simulink model "MSE_312_Electrical_Control_Model_The_Iron_Pirate"  (R2021a)
settings: Solver=ode15s  StartTime=0.0  StopTime=35  MaxStep=1  RelTol=1e-4  AbsTol=1e-4
libraries: fl_lib x15, nesl_utility x11, ee_lib x3, pid_lib x2
settings Model: Creator=junaidkhan  LastModifiedBy=Imad

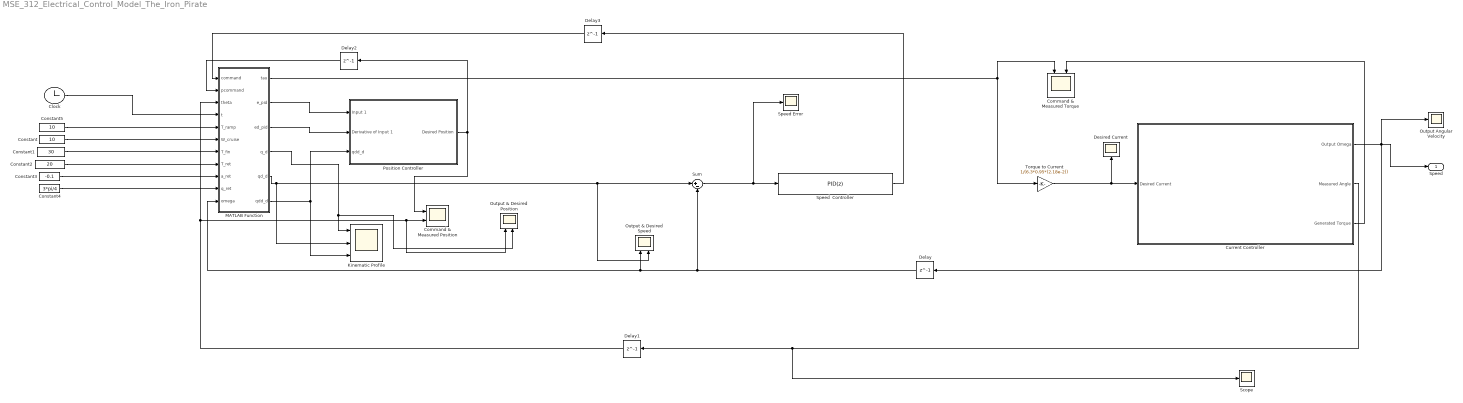
== system MSE_312_Electrical_Control_Model_The_Iron_Pirate ==
  " Output Angular Velocity" : Scope
  Clock : Clock
  Command & Measured Position : Scope  NumInputPorts=2
  Command & Measured Torque : Scope  NumInputPorts=2
  Constant : Constant  Value=10
  Constant1 : Constant  Value=30
  Constant2 : Constant  Value=20
  Constant3 : Constant  Value=-0.1
  Constant4 : Constant  Value=3*pi/4
  Constant5 : Constant  Value=10
  Current Controller : Subsystem
  Delay{,1..3} (4 alike) : Delay  DelayLength=1
  Desired Current : Scope
  Kinematic Profile : Scope  NumInputPorts=3
  MATLAB Function : MATLAB Function  TreatAsAtomicUnit=on
  Output & Desired Position : Scope  NumInputPorts=2
  Output & Desired Speed : Scope  NumInputPorts=2
  "Position Controller " : Subsystem
  Scope : Scope
  Speed  Controller : pid_lib/PID Controller  Controller=PID  Form=Ideal  TimeDomain=Discrete-time  UseExternalTs=off  SampleTime=1/4000  IntegratorMethod=Forward Euler  FilterMethod=Forward Euler  ControllerParametersSource=internal  P=1200*(0.00234)*(1/10)  I=0.0132  D=0.001  UseFilter=on  N=100  TunerSelectOption=Frequency Response Based  InitialConditionSource=internal  InitialConditionForIntegrator=0  InitialConditionForFilter=0  DifferentiatorICPrevScaledInput=0  ExternalReset=none  TrackingMode=off  Kt=1  LimitOutput=off  SatLimitsSource=internal  UpperSaturationLimit=inf  LowerSaturationLimit=-inf  LinearizeAsGain=on  AntiWindupMode=none  Kb=1  POutMin=[]  POutMax=[]  IOutMin=[]  IOutMax=[]  DOutMin=[]  DOutMax=[]  NOutMin=[]  NOutMax=[]  SumOutMin=[]  SumOutMax=[]  SaturationOutMin=[]  SaturationOutMax=[]  PParamMin=[]  PParamMax=[]  IParamMin=[]  IParamMax=[]  DParamMin=[]  DParamMax=[]  NParamMin=[]  NParamMax=[]  KbParamMin=[]  KbParamMax=[]  KtParamMin=[]  KtParamMax=[]  KbOutMin=[]  KbOutMax=[]  KtOutMin=[]  KtOutMax=[]  IntegratorOutMin=[]  IntegratorOutMax=[]  FilterOutMin=[]  FilterOutMax=[]  SumI1OutMin=[]  SumI1OutMax=[]  SumI2OutMin=[]  SumI2OutMax=[]  SumI3OutMin=[]  SumI3OutMax=[]  SumI4OutMin=[]  SumI4OutMax=[]  SumDOutMin=[]  SumDOutMax=[]  DifferentiatorOutMin=[]  DifferentiatorOutMax=[]  FilterDiffOutCoefMin=[]  FilterDiffOutCoefMax=[]  ReciprocalOutMin=[]  ReciprocalOutMax=[]  SumDenOutMin=[]  SumDenOutMax=[]  SumNumOutMin=[]  SumNumOutMax=[]  DivideOutMin=[]  DivideOutMax=[]  UdiffTsProdOutMin=[]  UdiffTsProdOutMax=[]  NTsProdOutMin=[]  NTsProdOutMax=[]  UintegralTsProdOutMin=[]  UintegralTsProdOutMax=[]  UngainTsProdOutMin=[]  UngainTsProdOutMax=[]  IntegratorContinuousStateAttributes=''  IntegratorStateMustResolveToSignalObject=off  IntegratorRTWStateStorageClass=Auto  FilterContinuousStateAttributes=''  FilterStateMustResolveToSignalObject=off  FilterRTWStateStorageClass=Auto  ParallelPVariant=Passthrough  IdealPVariant=InternalParameters  IVariant=InternalParameters  DVariant=InternalParameters  IntegratorVariant=Discrete  SatVariant=Disabled  AWVariant=Passthrough  PCopyVariant=Disabled  TRVariant=Disabled  FdbkBlocksVariant=Forward  IdealPFdbkVariant=Disabled  SatFdbkVariant=Disabled  DerivativeFilterVariant=ForwardEulerFilter  NVariant=InternalParameters  NCopyVariant=Disabled  FilterICVariant=InternalICsFilter  IntegratorICVariant=InternalICs  ExternalResetVariant=Disabled  TRSumVariant=Passthrough  SumFdbkVariant=Disabled  SumVariant=Sum_PID  TsampFilterVariant=InternalTs  TsampNgainVariant=Passthrough  TsampIntegralVariant=Passthrough  ExternalSaturationOutDataTypeStr=Inherit: Same as second input
  Speed Error : Scope
  Sum : Sum  Inputs=|+-
  Torque to Current : Gain  Gain=1/(6.3*0.95*(2.18e-2))
  Speed : Outport
  wires:
  Torque to Current/1 -> Current Controller/1("Desired Current "), Desired Current/1
  Speed  Controller/1 -> Delay3/1
  Sum/1 -> Speed Error/1, Speed  Controller/1
  Current Controller/3(Generated Torque) -> Command & Measured Torque/2
  MATLAB Function/5(qd_d) -> Sum/1, Output & Desired Speed/2, Kinematic Profile/2
  Delay/1 -> Sum/2, Output & Desired Speed/1, MATLAB Function/11(omega)
  Clock/1 -> MATLAB Function/4(t)
  Constant2/1 -> MATLAB Function/8(T_ret)
  Constant5/1 -> MATLAB Function/5(T_ramp)
  Constant3/1 -> MATLAB Function/9(a_ret)
  Constant4/1 -> MATLAB Function/10(q_ret)
  Constant/1 -> MATLAB Function/6(W_cruise)
  Constant1/1 -> MATLAB Function/7(T_fin)
  MATLAB Function/1(tau) -> Torque to Current/1, Command & Measured Torque/1
  Delay1/1 -> MATLAB Function/3(theta), Output & Desired Position/1, Command & Measured Position/2
  MATLAB Function/2(e_pid) -> "Position Controller "/1(Input 1)
  MATLAB Function/3(ed_pid) -> "Position Controller "/2(Derivative of Input 1)
  MATLAB Function/6(qdd_d) -> Kinematic Profile/3, "Position Controller "/3(qdd_d)
  MATLAB Function/4(q_d) -> Output & Desired Position/2, Kinematic Profile/1
  "Position Controller "/1(Desired Position) -> Command & Measured Position/1, Delay2/1
  Current Controller/1(Output Omega) -> Delay/1, Speed/1, " Output Angular Velocity"/1
  Current Controller/2("Measured Angle ") -> Scope/1, Delay1/1
  Delay2/1 -> MATLAB Function/2(pcommand)
  Delay3/1 -> MATLAB Function/1(command)

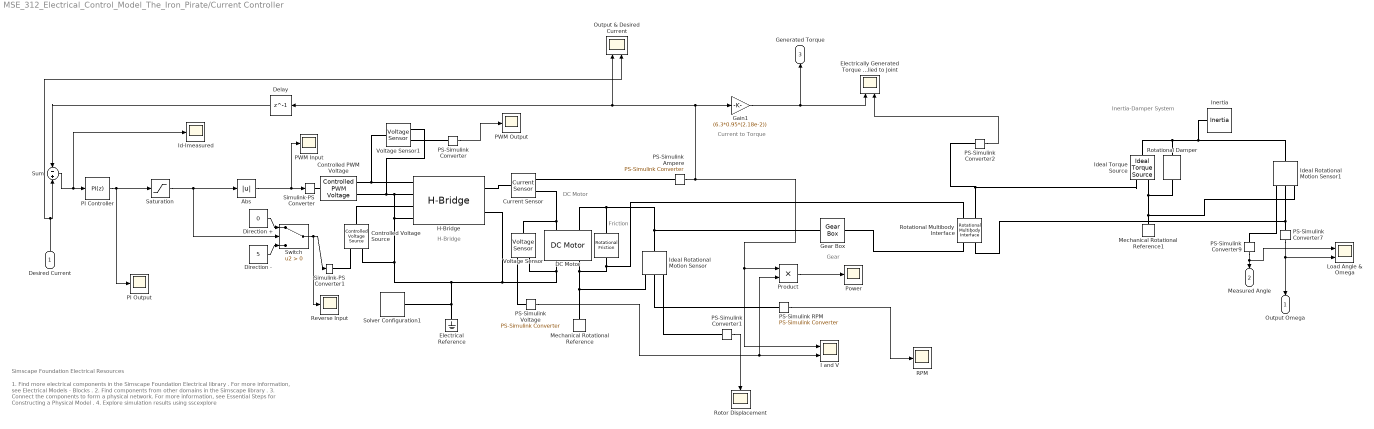
== system MSE_312_Electrical_Control_Model_The_Iron_Pirate/Current Controller ==
  note: Inertia-Damper System
  note: Current to Torque
  note: Gear
  note: H-Bridge
  note: DC Motor
  note: Friction
  note: 1. Find more electrical components in the Simscape Foundation Electrical library .
      | For more information, see Electrical Models - Blocks .
      | 2. Find components from other domains in the Simscape library .
      | 3. Connect the components to form a physical network.
      | For more information, see Essential Steps for Constructing a Physical Model .
      | 4. Explore simulation results using sscexplore
  note: Simscape Foundation Electrical Resources
  "Desired Current " : Inport
  " " : fl_lib/Mechanical/Rotational Elements/Rotational Friction  brkwy_trq=2.5e-3 N*m  brkwy_vel=0.1 rad/s  Col_trq=2.5e-3 N*m  visc_coef=0.001 N*m/(rad/s)  w_specify=off  w_priority=None  w=0 rad/s  w_nominal_specify=off  w_nominal_unit=rad/s  w_nominal_value=1  t_specify=off  t_priority=None  t=0 N*m  t_nominal_specify=off  t_nominal_unit=N*m  t_nominal_value=1
  Abs : Abs
  Controlled PWM Voltage : ee_lib/Integrated Circuits/Controlled PWM Voltage  F=4000 Hz  TD=0 s  pulse_width_offset=0 s  pulse_min=1 us  Vmin=0 V  Vmax=12 V  Vm=12 V  pwm_or_av=2  event_type=1  sample_time=1e-6 s  u_min=0  u_max=12
      settings: InternalSimscapePortConfiguration="{\"Bottom\":[],\"Left\":[{\"id\":\"u\",\"label\":\"u\",\"type\":\"input\"}],\"Right\":[{\"id\":\"p2\",\"label\":\"PWM\",\"type\":\"foundation.electrical.electrical\"},{\"id\":\"n2\",\"label\":\"REF\",\"type\":\"foundation.electrical.electrical\"}],\"Top\":[]}"
  Controlled Voltage Source : fl_lib/Electrical/Electrical Sources/Controlled Voltage Source
  Current Sensor : fl_lib/Electrical/Electrical Sensors/Current Sensor
  DC Motor : ee_lib/Electromechanical/Brushed Motors/DC Motor  field_option=ee.enum.field_option.pm  Rf=100 Ohm  Lf=1 H  Laf=0.15 H  If0=0 A  parameterization=ee.enum.dcparam_option.load_speed  Ra=4.33 Ohm  La=2.34 mH  emf_or_torque=ee.enum.emf_or_torque.kv  Kv=2.18e-2 V/rpm  Ki=6.876e-4 N*m/A  T_stall=3.0e-1 N*m  w_max=720 rpm  w_rated=350 rpm  P_rated=5.5 W  V_rated=12 V  J=1.6e-4 kg*m^2  lam_param=ee.enum.lam_param.current  lam=(1.114e-4) N*m/(rad/s)  i_noload=0.18 A  V_i_noload=12 V  speed0=0 rpm  enable_fault_armature=simscape.enum.onoff.off  rev_faulted=1 / 3  G_faulted_armature=1e-5 S  fault_trigger_armature=ee.enum.faults.faultTrigger.temporal  t_fault_armature=1 s  max_permissible_current_armature=inf A  t_fail_on_current_armature=1 s  enable_fault_field=simscape.enum.onoff.off  G_faulted_field=1e-5 S  fault_trigger_field=ee.enum.faults.faultTrigger.temporal  t_fault_field=1 s  max_permissible_current_field=inf A  t_fail_on_current_field=1 s  fault_action=simscape.enum.assert.action.none  alpha=3.93e-3 1/K  Tmeas=25 degC  thermal_mass=100 J/K  initial_temperature=25 degC
  Delay : Delay  DelayLength=1
  Direction + : Constant  Value=0
  Direction - : Constant  Value=5
  Electrical Reference : fl_lib/Electrical/Electrical Elements/Electrical Reference
  Electrically Generated Torque and Torque Applied to Joint : Scope  NumInputPorts=2
  Gain1 : Gain  Gain=(6.3*0.95*(2.18e-2))
  Gear Box : fl_lib/Mechanical/Mechanisms/Gear Box  ratio=1  t_in_specify=off  t_in_priority=None  t_in=0 N*m  t_in_nominal_specify=off  t_in_nominal_unit=N*m  t_in_nominal_value=1  t_out_specify=off  t_out_priority=None  t_out=0 N*m  t_out_nominal_specify=off  t_out_nominal_unit=N*m  t_out_nominal_value=1
      settings: LogSimulationData=on
  H-Bridge : ee_lib/Semiconductors & Converters/Converters/H-Bridge  supply_ports=ee.enum.supply_ports.hidesupply  Venable=2 V  Vmax=12 V  Vreverse=2.5 V  Vbrake=2.5 V  Vm=12 V  pwm_or_av=ee.enum.pwm_or_av.averaged  regenerative_braking_mode=ee.enum.converters.regenerative_braking_mode.depends_on_rev  discontinuous=ee.enum.current_profile.continuous  freewheeling_mode=ee.enum.converters.freewheeling_mode.two_diodes  Ron=0.55 Ohm  Don=1.3/3 Ohm  Goff=1e-6 S  Rload=10 Ohm  Lload=1e-5 H  F=10 kHz  thermal_mass=(1.25/298.15)*5 J/K  initial_temperature=298.15 K  Ron2=0.9 Ohm  Don2=1.7/3 Ohm  Tmeas=298.15 K  Tmeas2=360.65 K
  I and V : Scope  NumInputPorts=2
  Id-Imeasured : Scope
  Ideal Rotational Motion Sensor : fl_lib/Mechanical/Mechanical Sensors/Ideal Rotational Motion Sensor  wrap_angle=simscape.enum.onoff.off  offset=0 rad
  Ideal Rotational Motion Sensor1 : fl_lib/Mechanical/Mechanical Sensors/Ideal Rotational Motion Sensor  wrap_angle=simscape.enum.onoff.off  offset=0 rad
  Ideal Torque Source : fl_lib/Mechanical/Mechanical Sources/Ideal Torque Source
  Inertia : fl_lib/Mechanical/Rotational Elements/Inertia  inertia=8.3e-3 kg*m^2  num_ports=foundation.enum.numPorts2.one  w_specify=off  w_priority=High  w=0 rad/s  w_nominal_specify=off  w_nominal_unit=rad/s  w_nominal_value=1  t_specify=off  t_priority=None  t=0 N*m  t_nominal_specify=off  t_nominal_unit=N*m  t_nominal_value=1
  Load Angle & Omega : Scope  NumInputPorts=2
  Mechanical Rotational Reference : fl_lib/Mechanical/Rotational Elements/Mechanical Rotational Reference
  Mechanical Rotational Reference1 : fl_lib/Mechanical/Rotational Elements/Mechanical Rotational Reference
  Output & Desired Current : Scope  NumInputPorts=2
  PI Controller : pid_lib/PID Controller  Controller=PI  Form=Ideal  TimeDomain=Discrete-time  UseExternalTs=off  SampleTime=1/4000  IntegratorMethod=Forward Euler  FilterMethod=Forward Euler  ControllerParametersSource=internal  P=1200*(2.34e-3)  I=(120*4.33)/2  D=0  UseFilter=on  N=100  TunerSelectOption=Frequency Response Based  InitialConditionSource=internal  InitialConditionForIntegrator=0  InitialConditionForFilter=0  DifferentiatorICPrevScaledInput=0  ExternalReset=none  TrackingMode=off  Kt=1  LimitOutput=off  SatLimitsSource=internal  UpperSaturationLimit=inf  LowerSaturationLimit=-inf  LinearizeAsGain=on  AntiWindupMode=none  Kb=1  POutMin=[]  POutMax=[]  IOutMin=[]  IOutMax=[]  DOutMin=[]  DOutMax=[]  NOutMin=[]  NOutMax=[]  SumOutMin=[]  SumOutMax=[]  SaturationOutMin=[]  SaturationOutMax=[]  PParamMin=[]  PParamMax=[]  IParamMin=[]  IParamMax=[]  DParamMin=[]  DParamMax=[]  NParamMin=[]  NParamMax=[]  KbParamMin=[]  KbParamMax=[]  KtParamMin=[]  KtParamMax=[]  KbOutMin=[]  KbOutMax=[]  KtOutMin=[]  KtOutMax=[]  IntegratorOutMin=[]  IntegratorOutMax=[]  FilterOutMin=[]  FilterOutMax=[]  SumI1OutMin=[]  SumI1OutMax=[]  SumI2OutMin=[]  SumI2OutMax=[]  SumI3OutMin=[]  SumI3OutMax=[]  SumI4OutMin=[]  SumI4OutMax=[]  SumDOutMin=[]  SumDOutMax=[]  DifferentiatorOutMin=[]  DifferentiatorOutMax=[]  FilterDiffOutCoefMin=[]  FilterDiffOutCoefMax=[]  ReciprocalOutMin=[]  ReciprocalOutMax=[]  SumDenOutMin=[]  SumDenOutMax=[]  SumNumOutMin=[]  SumNumOutMax=[]  DivideOutMin=[]  DivideOutMax=[]  UdiffTsProdOutMin=[]  UdiffTsProdOutMax=[]  NTsProdOutMin=[]  NTsProdOutMax=[]  UintegralTsProdOutMin=[]  UintegralTsProdOutMax=[]  UngainTsProdOutMin=[]  UngainTsProdOutMax=[]  IntegratorContinuousStateAttributes=''  IntegratorStateMustResolveToSignalObject=off  IntegratorRTWStateStorageClass=Auto  FilterContinuousStateAttributes=''  FilterStateMustResolveToSignalObject=off  FilterRTWStateStorageClass=Auto  ParallelPVariant=Passthrough  IdealPVariant=InternalParameters  IVariant=InternalParameters  DVariant=Disabled  IntegratorVariant=Discrete  SatVariant=Disabled  AWVariant=Passthrough  PCopyVariant=Disabled  TRVariant=Disabled  FdbkBlocksVariant=Forward  IdealPFdbkVariant=Disabled  SatFdbkVariant=Disabled  DerivativeFilterVariant=Disabled  NVariant=Disabled  NCopyVariant=Disabled_SignalSpec  FilterICVariant=Disabled  IntegratorICVariant=InternalICs  ExternalResetVariant=Disabled  TRSumVariant=Passthrough  SumFdbkVariant=Disabled  SumVariant=Sum_PI  TsampFilterVariant=InternalTs  TsampNgainVariant=Passthrough  TsampIntegralVariant=Passthrough  ExternalSaturationOutDataTypeStr=Inherit: Same as second input
  PI Output : Scope
  PS-Simulink Ampere : nesl_utility/PS-Simulink Converter  PhysicalDomain=network_engine_domain  SubClassName=ps_output  LeftPortType=input  RightPortType=output  PseudoPeriodic=off  Frequencies=[]  Unit=A  AffineConversion=off
      settings: SourceProductBaseCode=PW,SS
  PS-Simulink Converter{,1..2,7,9} (5 alike) : nesl_utility/PS-Simulink Converter  PhysicalDomain=network_engine_domain  SubClassName=ps_output  LeftPortType=input  RightPortType=output  PseudoPeriodic=off  Frequencies=[]  Unit=inherit  AffineConversion=off
      settings: SourceProductBaseCode=PW,SS
  PS-Simulink RPM : nesl_utility/PS-Simulink Converter  PhysicalDomain=network_engine_domain  SubClassName=ps_output  LeftPortType=input  RightPortType=output  PseudoPeriodic=off  Frequencies=[]  Unit=rpm  AffineConversion=off
      settings: SourceProductBaseCode=PW,SS
  PS-Simulink Voltage : nesl_utility/PS-Simulink Converter  PhysicalDomain=network_engine_domain  SubClassName=ps_output  LeftPortType=input  RightPortType=output  PseudoPeriodic=off  Frequencies=[]  Unit=V  AffineConversion=off
      settings: SourceProductBaseCode=PW,SS
  PWM Input : Scope
  PWM Output : Scope
  Power : Scope
  Product : Product
  "RPM " : Scope
  Reverse Input : Scope
  Rotational Damper : fl_lib/Mechanical/Rotational Elements/Rotational Damper  D=0.0001 N*m/(rad/s)  w_specify=on  w_priority=None  w=0 rad/s  w_nominal_specify=off  w_nominal_unit=rad/s  w_nominal_value=1  t_specify=on  t_priority=None  t=0 N*m  t_nominal_specify=off  t_nominal_unit=N*m  t_nominal_value=1
  Rotational Multibody Interface : fl_lib/Mechanical/Multibody Interfaces/Rotational Multibody Interface
      settings: SourceProductBaseCode=SS
  Rotor Displacement : Scope
  Saturation : Saturate  UpperLimit=12  LowerLimit=-12
  Simulink-PS Converter : nesl_utility/Simulink-PS Converter  PhysicalDomain=network_engine_domain  SubClassName=ps_input  LeftPortType=input  RightPortType=output  PseudoPeriodic=off  Frequencies=[]  NoiseDistribution=none  NoiseParameters=[]  Unit=1  AffineConversion=off  FilteringAndDerivatives=provide  SimscapeFilterOrder=1  InputFilterTimeConstant=0.001  UdotUserProvided=0
      settings: SourceProductBaseCode=PW,SS
  Simulink-PS Converter1 : nesl_utility/Simulink-PS Converter  PhysicalDomain=network_engine_domain  SubClassName=ps_input  LeftPortType=input  RightPortType=output  PseudoPeriodic=off  Frequencies=[]  NoiseDistribution=none  NoiseParameters=[]  Unit=1  AffineConversion=off  FilteringAndDerivatives=provide  SimscapeFilterOrder=1  InputFilterTimeConstant=0.001  UdotUserProvided=0
      settings: SourceProductBaseCode=PW,SS
  Solver Configuration1 : nesl_utility/Solver Configuration  PhysicalDomain=network_engine_domain  SubClassName=solver  LeftPortType=input  RightPortType=generic  Tones=[]  Harmonics=[]  SimulateNoise=off  Profile=off  UseLocalSampling=off  EnableSwitchedLinearOptims=on  FrequencyDomain=off  UseCCode=off  RelTol=0.001  AbsTol=1e-06  MinStep=1e-09  ToWorkspace=off  RevertToSquareIcSolve=off  NumHomotopyIterations=100  PhasorMode=off  PhasorModeNumHarmonics=1  DoDC=off  ResidualTolerance=1e-09  UseLocalSolver=off  LocalSolverChoice=NE_BACKWARD_EULER_ADVANCER  LocalSolverSampleTime=0.001  DoFixedCost=off  MaxNonlinIter=3  MaxModeIter=2  ComputeImpulses=off  ImpulseIterations=2  LinearAlgebra=auto  EquationFormulation=NE_TIME_EF  DelaysMemoryBudget=1024  AutomaticFiltering=on  FilteringTimeConstant=0.001  PartitionStorageMethod=AS_NEEDED  PartitionMemoryBudget=1024  PartitionMethod=ROBUST
      settings: SourceProductBaseCode=PW,SS
  Sum : Sum  Inputs=-+
  Switch : Switch  Criteria=u2 > Threshold
  Voltage Sensor : fl_lib/Electrical/Electrical Sensors/Voltage Sensor
  Voltage Sensor1 : fl_lib/Electrical/Electrical Sensors/Voltage Sensor
  Output Omega : Outport
  "Measured Angle " : Outport  Port=2
  Generated Torque : Outport  Port=3
  wires:
  PS-Simulink Voltage/1 -> I and V/2, Product/2
  Switch/1 -> Reverse Input/1, Simulink-PS Converter1/1
  Sum/1 -> Id-Imeasured/1, PI Controller/1
  PS-Simulink Converter1/1 -> Rotor Displacement/1
  PS-Simulink Converter/1 -> PWM Output/1
  Abs/1 -> PWM Input/1, Simulink-PS Converter/1
  Product/1 -> Power/1
  Gain1/1 -> Generated Torque/1, Electrically Generated Torque and Torque Applied to Joint/1
  Direction +/1 -> Switch/1
  Direction -/1 -> Switch/3
  PI Controller/1 -> Saturation/1, PI Output/1
  PS-Simulink Converter2/1 -> Electrically Generated Torque and Torque Applied to Joint/2
  PS-Simulink RPM/1 -> "RPM "/1
  Saturation/1 -> Switch/2, Abs/1
  PS-Simulink Converter7/1 -> Output Omega/1, Load Angle & Omega/2
  PS-Simulink Converter9/1 -> Load Angle & Omega/1, "Measured Angle "/1
  PS-Simulink Ampere/1 -> Gain1/1, Delay/1, Output & Desired Current/1, I and V/1, Product/1
  Delay/1 -> Sum/1
  "Desired Current "/1 -> Output & Desired Current/2, Sum/2
  connections:
  PS-Simulink Converter/LConn1 -- Voltage Sensor1/RConn1
  PS-Simulink Voltage/LConn1 -- Voltage Sensor/RConn1
  Simulink-PS Converter/RConn1 -- Controlled PWM Voltage/LConn1
  PS-Simulink Converter1/LConn1 -- Ideal Rotational Motion Sensor/RConn3
  Controlled Voltage Source/LConn1 -- H-Bridge/LConn3
  H-Bridge/RConn1 -- Current Sensor/LConn1
  H-Bridge/LConn1 -- Controlled PWM Voltage/RConn1 -- Voltage Sensor1/LConn1
  DC Motor/LConn1 -- Voltage Sensor/LConn1 -- Current Sensor/RConn2
  Ideal Rotational Motion Sensor/RConn2 -- PS-Simulink RPM/LConn1
  Ideal Rotational Motion Sensor/RConn1 -- " "/LConn1 -- Rotational Multibody Interface/LConn2 -- DC Motor/RConn2 -- Mechanical Rotational Reference/LConn1
  Current Sensor/RConn1 -- PS-Simulink Ampere/LConn1
  H-Bridge/RConn2 -- Voltage Sensor/RConn2 -- DC Motor/RConn1 -- Voltage Sensor1/RConn2 -- Controlled PWM Voltage/RConn2 -- H-Bridge/LConn2 -- H-Bridge/LConn4 -- Controlled Voltage Source/RConn2 -- Electrical Reference/LConn1 -- Solver Configuration1/RConn1
  Simulink-PS Converter1/RConn1 -- Controlled Voltage Source/RConn1
  Gear Box/LConn1 -- Ideal Rotational Motion Sensor/LConn1 -- " "/RConn1 -- DC Motor/LConn2
  Gear Box/RConn1 -- Rotational Multibody Interface/RConn2
  PS-Simulink Converter2/LConn1 -- Ideal Torque Source/RConn1 -- Rotational Multibody Interface/LConn1
  Ideal Torque Source/LConn1 -- Rotational Damper/RConn1 -- Ideal Rotational Motion Sensor1/LConn1 -- Inertia/LConn1
  Ideal Torque Source/RConn2 -- Ideal Rotational Motion Sensor1/RConn1 -- Mechanical Rotational Reference1/LConn1 -- Rotational Damper/LConn1
  PS-Simulink Converter7/LConn1 -- Ideal Rotational Motion Sensor1/RConn2 -- Rotational Multibody Interface/RConn1
  Ideal Rotational Motion Sensor1/RConn3 -- PS-Simulink Converter9/LConn1

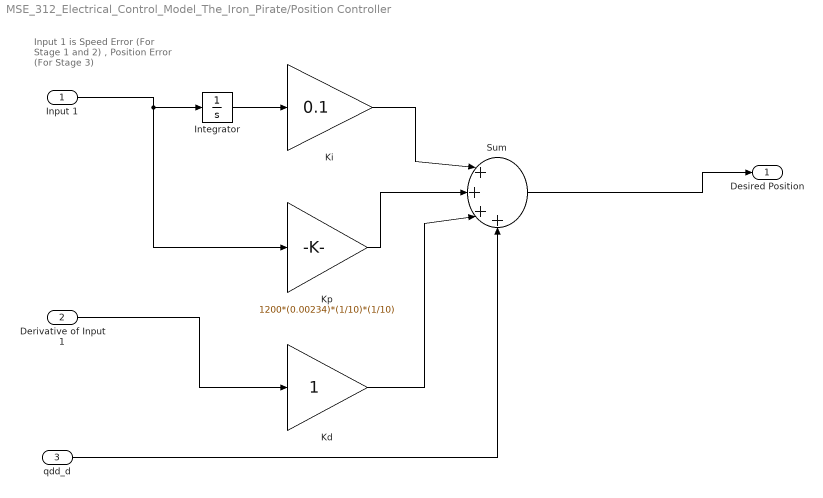
== system MSE_312_Electrical_Control_Model_The_Iron_Pirate/Position Controller  ==
  note: Input 1 is Speed Error
      | (For Stage 1 and 2)
      | , Position Error
      | (For Stage 3)
  Input 1 : Inport
  Derivative of Input 1 : Inport  Port=2
  qdd_d : Inport  Port=3
  Integrator : Integrator
  Kd : Gain
  Ki : Gain  Gain=0.1
  Kp : Gain  Gain=1200*(0.00234)*(1/10)*(1/10)
  Sum : Sum  Inputs=|++++
  Desired Position : Outport
  wires:
  Ki/1 -> Sum/1
  qdd_d/1 -> Sum/4
  Integrator/1 -> Ki/1
  Kd/1 -> Sum/3
  Derivative of Input 1/1 -> Kd/1
  Input 1/1 -> Kp/1, Integrator/1
  Kp/1 -> Sum/2
  Sum/1 -> Desired Position/1

== matlab function MSE_312_Electrical_Control_Model_The_Iron_Pirate/MATLAB Function ==
  data: command input; tau output; pcommand input; theta input; t input; T_ramp input; W_cruise input; T_fin input; T_ret input; a_ret input; q_ret input; omega input; e_pid output; ed_pid output; q_d output; qd_d output; qdd_d output
function [tau, e_pid, ed_pid, q_d, qd_d, qdd_d] = fcn(command, pcommand, theta, t, T_ramp, W_cruise, T_fin, T_ret, a_ret, q_ret, omega)
    
    if (t <= T_ramp)
        q_d = 0.5 * W_cruise * t^2/T_ramp;
        qd_d = W_cruise * t/T_ramp;
        qdd_d = W_cruise/T_ramp;
        e_pid = qd_d - omega;
        tau = command;
        q_0 = []; q_1 = []; q_2 = []; q_3 = []; ed_pid = 0;

    elseif (t > T_ramp && t < T_ret)
        q_d = 0.5 * W_cruise * T_ramp + W_cruise * (t-T_ramp);
        qd_d = W_cruise;
        qdd_d = 0;
        e_pid = qd_d - omega;
        tau = command;
        q_0 = []; q_1 = []; q_2 = []; q_3 = []; q_4 = []; q_5 = []; ed_pid = 0;

    elseif (t >= T_ret && t < T_fin)
        De1 = T_fin - T_ret;
        q_2 = a_ret * 0.5;
        q_1 = W_cruise;
        %q_0 = q_ret;
        %q_0 = 0.5*(W_cruise/T_ramp)*(T_ramp*2) + W_cruise*(T_ramp);
        q_0 = 150;
        ii = inv([De1^3 De1^4 De1^5; 3*De1^2 4*De1^3 5*De1^4; 6*De1 12*De1^2 20*De1^3])*([-q_0-q_1*De1-q_2*De1^2; -q_1-2*q_2*De1; -2*q_2]);
        q_3 = ii(1); q_4 = ii(2); q_5 = ii(3);
        De1_T = t - T_ret;

        q_d = q_0 + q_1*De1_T +q_2*De1_T^2 + q_3*De1_T^3 + q_4*De1_T^4 + q_5*De1_T^5;
        qd_d = q_1 + 2*q_2*De1_T + 3*q_3*De1_T^2 + 4*q_4*De1_T^3 + 5*q_5*De1_T^4;
        qdd_d = 2*q_2 + 6*q_3*De1_T + 12*q_4*De1_T^2 + 20*q_5*De1_T^3;
        e_pid = q_d - theta;
        ed_pid = qd_d - omega;
        tau = pcommand;

    else
        q_d = 0;
        qd_d = 0;
        qdd_d = 0;
        e_pid = q_d - theta;
        ed_pid = qd_d - omega;
        tau = pcommand;
    end
end
